simulink model "TwoDOFRobotDynCon"  (R2013b)
settings: Solver=ode45  StartTime=0.0  StopTime=10  RelTol=1e-3
libraries: simulink x2
settings Model: Creator=Ahsan  LastModifiedBy=Ahsan

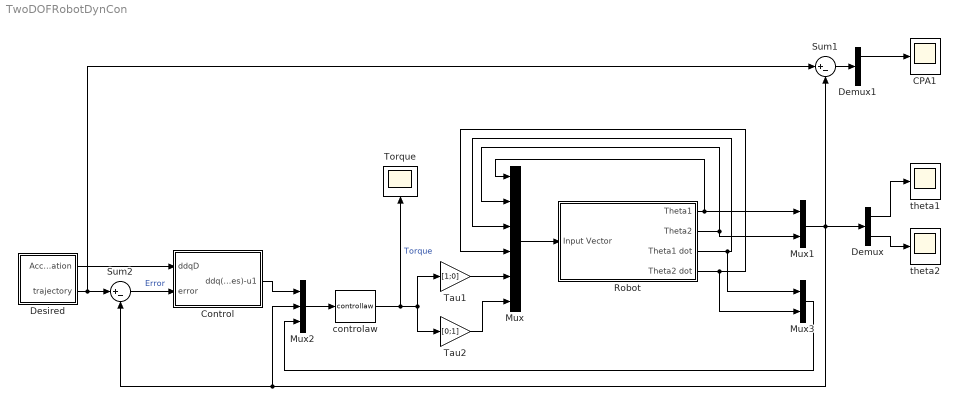
== system TwoDOFRobotDynCon ==
  CPA1 : Scope
      settings: YMin=-1400  YMax=100  SaveName=ScopeData4
  Control : Subsystem
  Demux : Demux  Outputs=2
  Demux1 : Demux  Outputs=2
  "Desired " : Subsystem
  Mux : Mux  Inputs=6
  Mux1 : Mux  Inputs=2
  Mux2 : Mux  Inputs=3
  Mux3 : Mux  Inputs=2
  Robot : Subsystem
  Sum1 : Sum  Inputs=|+-
  Sum2 : Sum  Inputs=|+-
  Tau1 : Gain  Gain=[1;0]
  Tau2 : Gain  Gain=[0;1]
  Torque : Scope
  controlaw : MATLABFcn  MATLABFcn=controllaw  OutputDimensions=2
  theta1 : Scope
      settings: YMin=-50000  YMax=-7500  SaveName=ScopeData2
  theta2 : Scope
      settings: YMin=0  YMax=10000
  wires:
  Mux/1 -> Robot/1(Input Vector)
  Robot/1("Theta1 ") -> Mux1/1, Mux/1
  Robot/2(Theta2) -> Mux1/2, Mux/2
  Robot/3(Theta1 dot) -> Mux3/1, Mux/3
  Robot/4(Theta2 dot) -> Mux3/2, Mux/4
  Mux1/1 -> Demux/1, Sum1/2, Sum2/2, Mux2/2
  Tau1/1 -> Mux/5
  Tau2/1 -> Mux/6
  Sum2/1 -> Control/2(error)  "Error"
  Mux2/1 -> controlaw/1
  controlaw/1 -> Tau2/1, Tau1/1, Torque/1  "Torque"
  Mux3/1 -> Mux2/3
  Control/1(ddq(des)-u1) -> Mux2/1
  Demux/1 -> theta1/1
  Demux/2 -> theta2/1
  "Desired "/2(trajectory) -> Sum2/1, Sum1/1
  Sum1/1 -> Demux1/1
  Demux1/1 -> CPA1/1
  "Desired "/1(Acceleration) -> Control/1(ddqD)

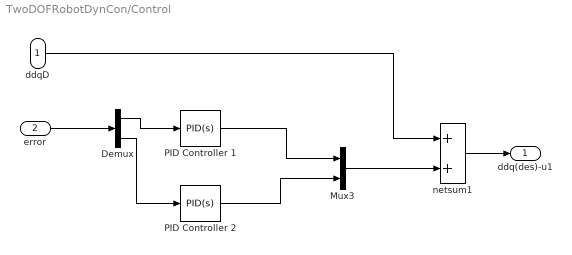
== system TwoDOFRobotDynCon/Control ==
  ddqD : Inport
  error : Inport  Port=2
  Demux : Demux  Outputs=2
  Mux3 : Mux  Inputs=2
  PID Controller 1 : simulink/Continuous/PID Controller  Controller=PID  TimeDomain=Continuous-time  SampleTime=1  IntegratorMethod=Forward Euler  FilterMethod=Forward Euler  Form=Parallel  P=1500  I=800  D=3000  N=287.53756707028  InitialConditionSource=internal  InitialConditionForIntegrator=0  InitialConditionForFilter=0  ExternalReset=none  LimitOutput=off  UpperSaturationLimit=inf  LowerSaturationLimit=-inf  LinearizeAsGain=on  AntiWindupMode=none  Kb=1  TrackingMode=off  Kt=1  PParamMin=[]  PParamMax=[]  IParamMin=[]  IParamMax=[]  DParamMin=[]  DParamMax=[]  NParamMin=[]  NParamMax=[]  KbParamMin=[]  KbParamMax=[]  KtParamMin=[]  KtParamMax=[]  POutMin=[]  POutMax=[]  IOutMin=[]  IOutMax=[]  DOutMin=[]  DOutMax=[]  NOutMin=[]  NOutMax=[]  KbOutMin=[]  KbOutMax=[]  KtOutMin=[]  KtOutMax=[]  IntegratorOutMin=[]  IntegratorOutMax=[]  FilterOutMin=[]  FilterOutMax=[]  SumOutMin=[]  SumOutMax=[]  SumI1OutMin=[]  SumI1OutMax=[]  SumI2OutMin=[]  SumI2OutMax=[]  SumI3OutMin=[]  SumI3OutMax=[]  SumDOutMin=[]  SumDOutMax=[]  SaturationOutMin=[]  SaturationOutMax=[]  IntegratorContinuousStateAttributes=''  IntegratorStateMustResolveToSignalObject=off  IntegratorRTWStateStorageClass=Auto  FilterContinuousStateAttributes=''  FilterStateMustResolveToSignalObject=off  FilterRTWStateStorageClass=Auto
  PID Controller 2 : simulink/Continuous/PID Controller  Controller=PID  TimeDomain=Continuous-time  SampleTime=1  IntegratorMethod=Forward Euler  FilterMethod=Forward Euler  Form=Parallel  P=1  I=1  D=1  N=1  InitialConditionSource=internal  InitialConditionForIntegrator=0  InitialConditionForFilter=0  ExternalReset=none  LimitOutput=off  UpperSaturationLimit=inf  LowerSaturationLimit=-inf  LinearizeAsGain=on  AntiWindupMode=none  Kb=1  TrackingMode=off  Kt=1  PParamMin=[]  PParamMax=[]  IParamMin=[]  IParamMax=[]  DParamMin=[]  DParamMax=[]  NParamMin=[]  NParamMax=[]  KbParamMin=[]  KbParamMax=[]  KtParamMin=[]  KtParamMax=[]  POutMin=[]  POutMax=[]  IOutMin=[]  IOutMax=[]  DOutMin=[]  DOutMax=[]  NOutMin=[]  NOutMax=[]  KbOutMin=[]  KbOutMax=[]  KtOutMin=[]  KtOutMax=[]  IntegratorOutMin=[]  IntegratorOutMax=[]  FilterOutMin=[]  FilterOutMax=[]  SumOutMin=[]  SumOutMax=[]  SumI1OutMin=[]  SumI1OutMax=[]  SumI2OutMin=[]  SumI2OutMax=[]  SumI3OutMin=[]  SumI3OutMax=[]  SumDOutMin=[]  SumDOutMax=[]  SaturationOutMin=[]  SaturationOutMax=[]  IntegratorContinuousStateAttributes=''  IntegratorStateMustResolveToSignalObject=off  IntegratorRTWStateStorageClass=Auto  FilterContinuousStateAttributes=''  FilterStateMustResolveToSignalObject=off  FilterRTWStateStorageClass=Auto
  netsum1 : Sum  Inputs=2  SaturateOnIntegerOverflow=on  InputSameDT=on  OutDataTypeStr=Inherit: Same as first input
  ddq(des)-u1 : Outport
  wires:
  ddqD/1 -> netsum1/1
  error/1 -> Demux/1
  Demux/2 -> PID Controller 2/1
  Demux/1 -> PID Controller 1/1
  PID Controller 1/1 -> Mux3/1
  PID Controller 2/1 -> Mux3/2
  Mux3/1 -> netsum1/2
  netsum1/1 -> ddq(des)-u1/1

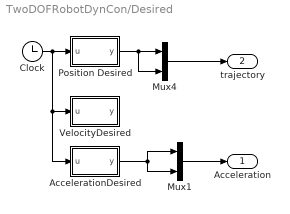
== system TwoDOFRobotDynCon/Desired  ==
  AccelerationDesired : MATLAB Function  TreatAsAtomicUnit=on
  Clock : Clock
  Mux1 : Mux  Inputs=2
  Mux4 : Mux  Inputs=2
  Position Desired : MATLAB Function  TreatAsAtomicUnit=on
  VelocityDesired : MATLAB Function  TreatAsAtomicUnit=on
  Acceleration : Outport
  trajectory : Outport  Port=2
  wires:
  Position Desired/1(y) -> Mux4/1, Mux4/2
  Clock/1 -> AccelerationDesired/1(u), VelocityDesired/1(u), Position Desired/1(u)
  Mux4/1 -> trajectory/1
  AccelerationDesired/1(y) -> Mux1/1, Mux1/2
  Mux1/1 -> Acceleration/1

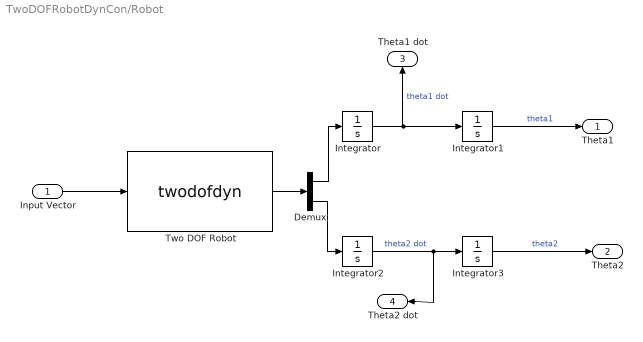
== system TwoDOFRobotDynCon/Robot ==
  Input Vector : Inport
  Demux : Demux  Outputs=2
  Integrator{,1..3} (4 alike) : Integrator
  Two DOF Robot : MATLABFcn  MATLABFcn=twodofdyn  OutputDimensions=2
  "Theta1 " : Outport
  Theta2 : Outport  Port=2
  Theta1 dot : Outport  Port=3
  Theta2 dot : Outport  Port=4
  wires:
  Two DOF Robot/1 -> Demux/1
  Input Vector/1 -> Two DOF Robot/1
  Integrator/1 -> Theta1 dot/1, Integrator1/1  "theta1 dot"
  Demux/1 -> Integrator/1
  Integrator2/1 -> Theta2 dot/1, Integrator3/1  "theta2 dot"
  Integrator3/1 -> Theta2/1  "theta2"
  Integrator1/1 -> "Theta1 "/1  "theta1"
  Demux/2 -> Integrator2/1

== matlab function TwoDOFRobotDynCon/Desired /Position Desired ==
  data: u input; y output
function y = fcn(u)
%#codegen

y =1-cos(pi*u);

== matlab function TwoDOFRobotDynCon/Desired /AccelerationDesired ==
  data: u input; y output
function y = fcn(u)
%#codegen

y =pi*pi*cos(pi*u);

== matlab function TwoDOFRobotDynCon/Desired /VelocityDesired ==
  data: u input; y output
function y = fcn(u)
%#codegen

y =pi*sin(pi*u);
